simulink model "chapter_3_homework"  (R2022a)
settings: Solver=VariableStepAuto  StartTime=0.0  StopTime=100  RelTol=1e-3
settings Model: Creator=slack  LastModifiedBy=slack

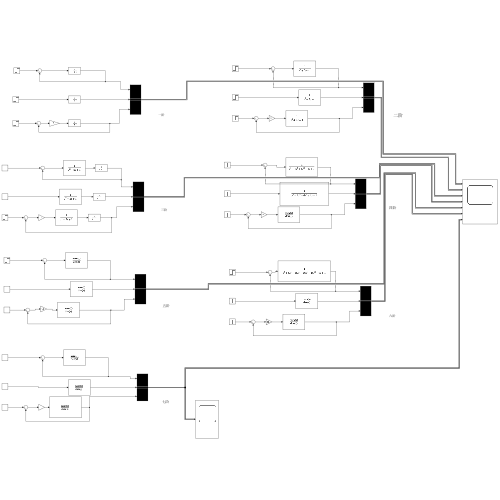
[thumbnail: Simulink's stored preview of the top-level diagram]
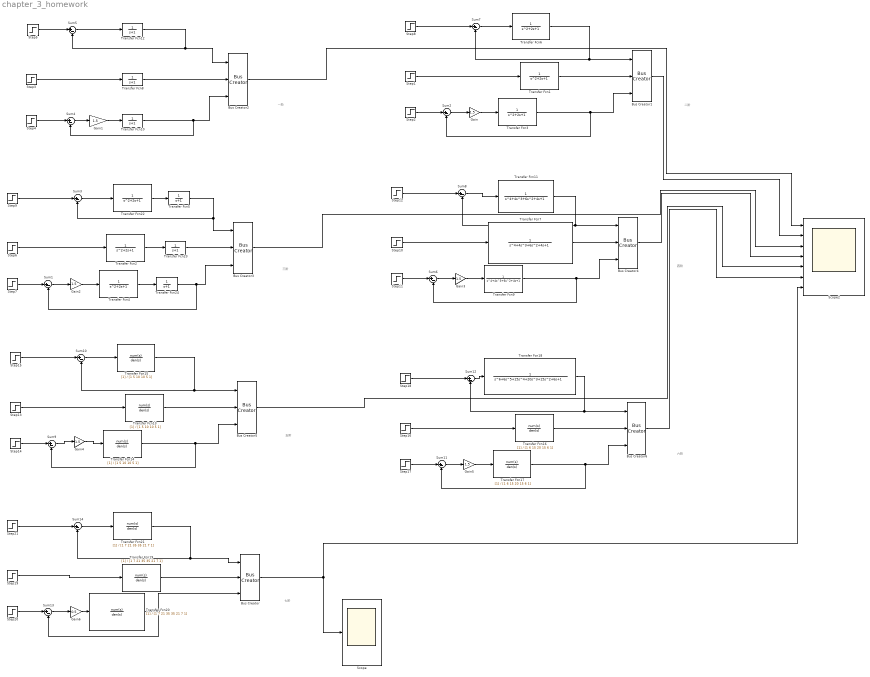
== system chapter_3_homework ==
  note: 七阶
  note: 六阶
  note: 五阶
  note: 四阶
  note: 三阶
  note: 二阶
  note: 一阶
  Bus Creator{,1..6} (7 alike) : BusCreator  Inputs=3
  Gain{,1..5} (6 alike) : Gain  Gain=1.5
  Gain6 : Gain  Gain=0.5
  Scope : Scope
  Scope2 : Scope  NumInputPorts=7
  Step{1,3,5..6,8..10,12..13,15..16,18..19,21} (14 alike) : Step  After=2  SampleTime=0
  Step{2,4,7,11,14,17,20} (7 alike) : Step  SampleTime=0
  Sum{1..14} (14 alike) : Sum  Inputs=|+-
  Transfer Fcn{1..4,6,22} (6 alike) : TransferFcn
  Transfer Fcn{5,8,10,12,23..24} (6 alike) : TransferFcn  Denominator=[1 1]
  Transfer Fcn11 : TransferFcn  Denominator=[1 4 6 4 1]
  Transfer Fcn13 : TransferFcn  Denominator=[1 5 10 10 5 1]
  Transfer Fcn14 : TransferFcn  Denominator=[1 5 10 10 5 1]
  Transfer Fcn15 : TransferFcn  Denominator=[1 5 10 10 5 1]
  Transfer Fcn16 : TransferFcn  Denominator=[1 6 15 20 15 6 1]
  Transfer Fcn17 : TransferFcn  Denominator=[1 6 15 20 15 6 1]
  Transfer Fcn18 : TransferFcn  Denominator=[1 6 15 20 15 6 1]
  Transfer Fcn19 : TransferFcn  Denominator=[1 7 21 35 35 21 7 1]
  Transfer Fcn20 : TransferFcn  Denominator=[1 7 21 35 35 21 7 1]
  Transfer Fcn21 : TransferFcn  Denominator=[1 7 21 35 35 21 7 1]
  Transfer Fcn7 : TransferFcn  Denominator=[1 4 6 4 1]
  Transfer Fcn9 : TransferFcn  Denominator=[1 4 6 4 1]
  wires:
  Sum7/1 -> Transfer Fcn6/1
  Transfer Fcn6/1 -> Sum7/2, Bus Creator1/1
  Bus Creator1/1 -> Scope2/2
  Step8/1 -> Sum7/1
  Step1/1 -> Transfer Fcn1/1
  Transfer Fcn1/1 -> Bus Creator1/2
  Step2/1 -> Sum2/1
  Transfer Fcn3/1 -> Bus Creator1/3, Sum2/2
  Sum2/1 -> Gain/1
  Gain/1 -> Transfer Fcn3/1
  Gain1/1 -> Transfer Fcn10/1
  Step3/1 -> Transfer Fcn8/1
  Transfer Fcn8/1 -> Bus Creator2/2
  Step5/1 -> Sum5/1
  Step4/1 -> Sum4/1
  Transfer Fcn12/1 -> Sum5/2, Bus Creator2/1
  Transfer Fcn10/1 -> Bus Creator2/3, Sum4/2
  Bus Creator2/1 -> Scope2/1
  Sum5/1 -> Transfer Fcn12/1
  Sum4/1 -> Gain1/1
  Gain2/1 -> Transfer Fcn4/1
  Step9/1 -> Sum3/1
  Step7/1 -> Sum1/1
  Bus Creator3/1 -> Scope2/3
  Sum3/1 -> Transfer Fcn22/1
  Sum1/1 -> Gain2/1
  Transfer Fcn11/1 -> Sum8/2, Bus Creator4/1
  Step10/1 -> Transfer Fcn7/1
  Transfer Fcn9/1 -> Bus Creator4/3, Sum6/2
  Gain3/1 -> Transfer Fcn9/1
  Step12/1 -> Sum8/1
  Step11/1 -> Sum6/1
  Transfer Fcn7/1 -> Bus Creator4/2
  Sum8/1 -> Transfer Fcn11/1
  Sum6/1 -> Gain3/1
  Transfer Fcn15/1 -> Sum10/2, Bus Creator5/1
  Step13/1 -> Transfer Fcn13/1
  Transfer Fcn14/1 -> Bus Creator5/3, Sum9/2
  Gain4/1 -> Transfer Fcn14/1
  Step15/1 -> Sum10/1
  Step14/1 -> Sum9/1
  Transfer Fcn13/1 -> Bus Creator5/2
  Sum10/1 -> Transfer Fcn15/1
  Sum9/1 -> Gain4/1
  Transfer Fcn18/1 -> Sum12/2, Bus Creator6/1
  Step16/1 -> Transfer Fcn16/1
  Transfer Fcn17/1 -> Bus Creator6/3, Sum11/2
  Gain5/1 -> Transfer Fcn17/1
  Step18/1 -> Sum12/1
  Step17/1 -> Sum11/1
  Bus Creator6/1 -> Scope2/6
  Transfer Fcn16/1 -> Bus Creator6/2
  Sum12/1 -> Transfer Fcn18/1
  Sum11/1 -> Gain5/1
  Transfer Fcn21/1 -> Bus Creator/1, Sum14/2
  Step19/1 -> Transfer Fcn19/1
  Transfer Fcn20/1 -> Bus Creator/3, Sum13/2
  Gain6/1 -> Transfer Fcn20/1
  Step21/1 -> Sum14/1
  Step20/1 -> Sum13/1
  Bus Creator/1 -> Scope2/7, Scope/1
  Sum14/1 -> Transfer Fcn21/1
  Sum13/1 -> Gain6/1
  Transfer Fcn22/1 -> Transfer Fcn5/1
  Transfer Fcn5/1 -> Sum3/2, Bus Creator3/1
  Step6/1 -> Transfer Fcn2/1
  Transfer Fcn2/1 -> Transfer Fcn23/1
  Transfer Fcn4/1 -> Transfer Fcn24/1
  Transfer Fcn24/1 -> Bus Creator3/3, Sum1/2
  Bus Creator4/1 -> Scope2/4
  Bus Creator5/1 -> Scope2/5
  Transfer Fcn19/1 -> Bus Creator/2
  Transfer Fcn23/1 -> Bus Creator3/2
